simulink model "weather_demo"  (Simulink 8.1)
settings: Solver=FixedStepDiscrete  StartTime=0.0  StopTime=8760*3600  FixedStep=3600  RelTol=1e-3
libraries: CampusModeling x1
settings Model: Creator=sfrank1  LastModifiedBy=sfrank1
settings DataIOCC: SignalLoggingSaveFormat=Dataset
settings OptimizationCC: ExpressionDepthLimit=128
settings DebuggingCC: FcnCallInpInsideContextMsg=EnableAllAsError
settings GRTTargetCC: CombineOutputUpdateFcns=on  GRTInterface=off

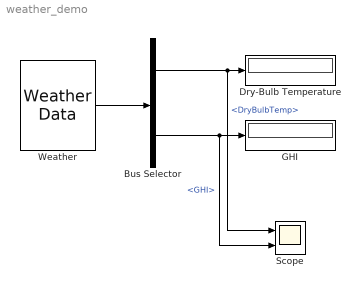
== system weather_demo ==
  Bus Selector : BusSelector  OutputSignals=DryBulbTemp,GHI
  Dry-Bulb Temperature : Display
  GHI : Display
  Scope : Scope  NumInputPorts=2
      settings: YMin=-5~-5  YMax=5~5
  Weather : CampusModeling/Weather/Weather Data  fname=TMY3.mat  initbus=on
  wires:
  Bus Selector/1 -> Scope/1, Dry-Bulb Temperature/1  "<DryBulbTemp>"
  Bus Selector/2 -> Scope/2, GHI/1  "<GHI>"
  Weather/1 -> Bus Selector/1
